simulink subsystem "LaneChangeMetrics"  (R2024b)
settings: Solver=VariableStepAuto  StartTime=0.0  StopTime=10.0  RelTol=1e-3
undefined symbols (not defined in the file): assessment, mapInfo
libraries: simulink x5
settings Model: Creator=The MathWorks, Inc.  LastModifiedBy=The MathWorks, Inc.
settings SolverCC: MaxZcPerStep=1
settings DebuggingCC: UnconnectedInputMsg=warning  UnconnectedOutputMsg=warning  UnconnectedLineMsg=warning  SubsystemReferenceDiagnosticForUnitTest=warning
settings ModelReferenceCC: EnableRefExpFcnMdlSchedulingChecks=on
settings RTWCC: GPUComputeCapability=3.5  DLArmComputeVersion=19.05

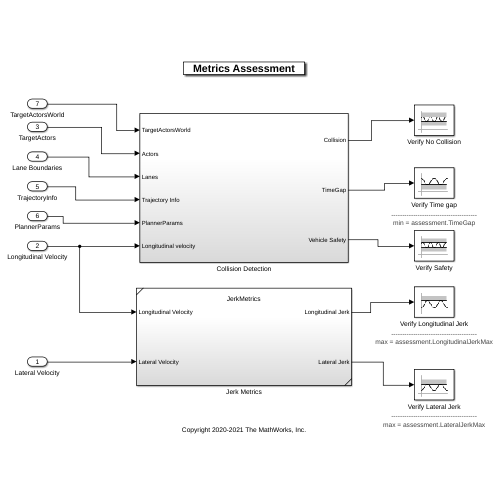
[thumbnail: Simulink's stored preview of the top-level diagram]
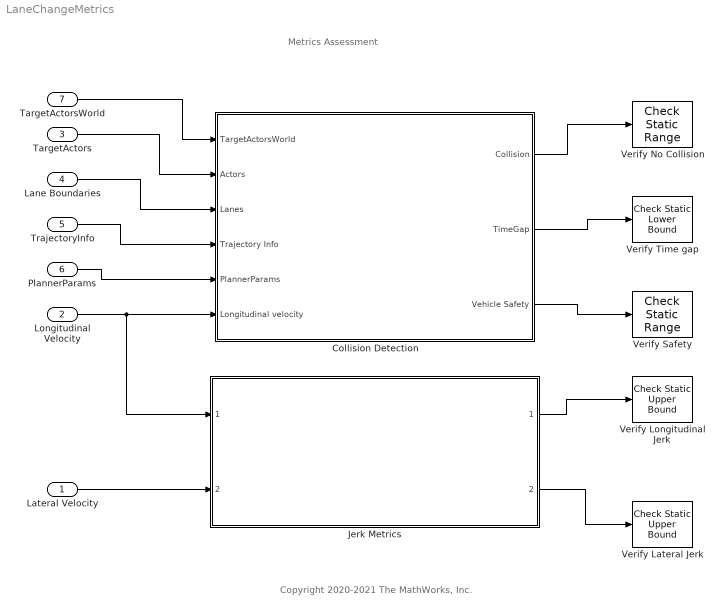
== system LaneChangeMetrics ==
  note: Metrics Assessment
  note: Copyright 2020-2021 The MathWorks, Inc.
  Lateral Velocity : Inport
  Longitudinal Velocity : Inport  Port=2
  TargetActors : Inport  Port=3
  Lane Boundaries : Inport  Port=4
  TrajectoryInfo : Inport  Port=5
  PlannerParams : Inport  Port=6
  TargetActorsWorld : Inport  Port=7
  Collision Detection : Subsystem
  Jerk Metrics : Subsystem  ReferencedSubsystem=JerkMetrics
  Verify Lateral Jerk : simulink/Model Verification/Check Static  Upper Bound  Description=u <= assessment.LateralJerkMax  max=assessment.LateralJerkMax  max_included=on  enabled=on  stopWhenAssertionFail=off  export=off  icon=graphic
      settings: AttributesFormatString=|
      | ---------------------------------------
      | max = %<max>
  Verify Longitudinal Jerk : simulink/Model Verification/Check Static  Upper Bound  Description=u <= assessment.LongitudinalJerkMax  max=assessment.LongitudinalJerkMax  max_included=on  enabled=on  stopWhenAssertionFail=off  export=off  icon=graphic
      settings: AttributesFormatString=|
      | ---------------------------------------
      | max = %<max>
  Verify No Collision : simulink/Model Verification/Check  Static Range  Description=0 <= u <= 0  max=0  max_included=on  min=0  min_included=on  enabled=on  stopWhenAssertionFail=on  export=off  icon=graphic
  Verify Safety : simulink/Model Verification/Check  Static Range  Description=1 <= u <= 1  max=1  max_included=on  min=1  min_included=on  enabled=on  stopWhenAssertionFail=off  export=off  icon=graphic
  Verify Time gap : simulink/Model Verification/Check Static  Lower Bound  Description=assessment.TimeGap <= u  min=assessment.TimeGap  min_included=on  enabled=on  stopWhenAssertionFail=off  export=off  icon=graphic
      settings: AttributesFormatString=|
      | ---------------------------------------
      | min = %<min>
  wires:
  Lateral Velocity/1 -> Jerk Metrics/2
  Jerk Metrics/1 -> Verify Longitudinal Jerk/1
  Jerk Metrics/2 -> Verify Lateral Jerk/1
  TargetActors/1 -> Collision Detection/2(Actors)
  Lane Boundaries/1 -> Collision Detection/3(Lanes)
  Collision Detection/3(Vehicle Safety) -> Verify Safety/1
  Collision Detection/2(TimeGap) -> Verify Time gap/1
  TrajectoryInfo/1 -> Collision Detection/4(Trajectory Info)
  Collision Detection/1(Collision) -> Verify No Collision/1
  PlannerParams/1 -> Collision Detection/5(PlannerParams)
  Longitudinal Velocity/1 -> Collision Detection/6(Longitudinal velocity), Jerk Metrics/1
  TargetActorsWorld/1 -> Collision Detection/1(TargetActorsWorld)

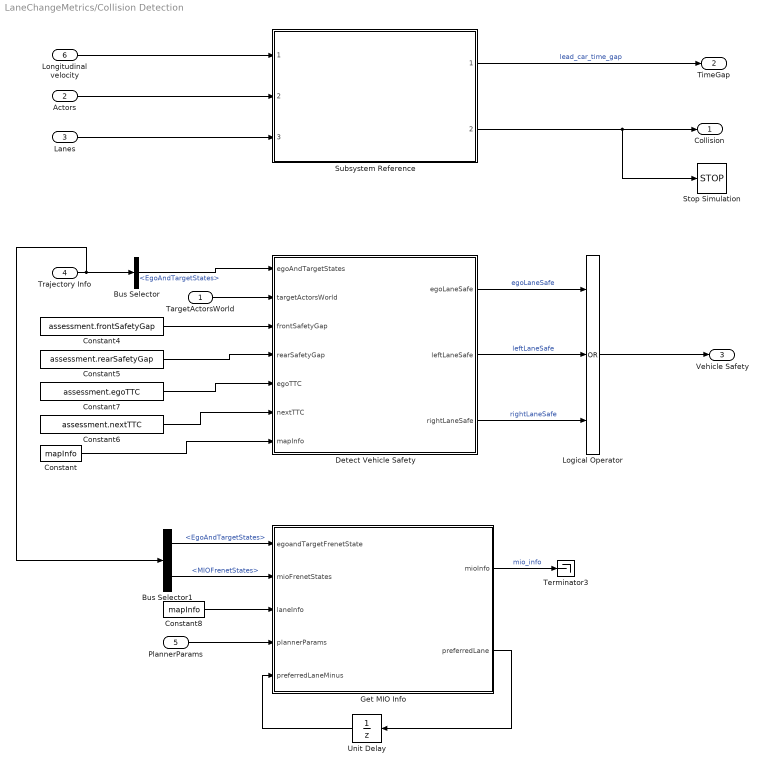
== system LaneChangeMetrics/Collision Detection ==
  TargetActorsWorld : Inport
  Actors : Inport  Port=2
  Lanes : Inport  Port=3
  Trajectory Info : Inport  Port=4
  PlannerParams : Inport  Port=5
  Longitudinal velocity : Inport  Port=6
  Bus Selector : BusSelector  OutputSignals=EgoAndTargetStates
  Bus Selector1 : BusSelector  OutputSignals=EgoAndTargetStates,MIOFrenetStates
  Constant : Constant  Value=mapInfo  OutDataTypeStr=Bus: BusMapInfo
  Constant4 : Constant  Value=assessment.frontSafetyGap
  Constant5 : Constant  Value=assessment.rearSafetyGap
  Constant6 : Constant  Value=assessment.nextTTC
  Constant7 : Constant  Value=assessment.egoTTC
  Constant8 : Constant  Value=mapInfo  OutDataTypeStr=Bus: BusMapInfo
  Detect Vehicle Safety : MATLAB Function  TreatAsAtomicUnit=on
  Get MIO Info : MATLAB Function  TreatAsAtomicUnit=on  mask{outputStructObj=Simulink.Bus.createMATLABStruct('BusMIOInfo')}
      mask prompts: outputStructObj "Output Structure"
  Logical Operator : Logic  Operator=OR  Inputs=3  AllPortsSameDT=off  OutDataTypeStr=boolean
  Stop Simulation : Stop
  Subsystem Reference : Subsystem  ReferencedSubsystem=CollisionDetection
  Terminator3 : Terminator
  Unit Delay : UnitDelay  SampleTime=-1  HasFrameUpgradeWarning=on
  Collision : Outport
  TimeGap : Outport  Port=2
  Vehicle Safety : Outport  Port=3
  wires:
  TargetActorsWorld/1 -> Detect Vehicle Safety/2(targetActorsWorld)
  Constant8/1 -> Get MIO Info/3(laneInfo)
  Bus Selector1/2 -> Get MIO Info/2(mioFrenetStates)  "<MIOFrenetStates>"
  Trajectory Info/1 -> Bus Selector/1, Bus Selector1/1
  Bus Selector1/1 -> Get MIO Info/1(egoandTargetFrenetState)  "<EgoAndTargetStates>"
  Unit Delay/1 -> Get MIO Info/5(preferredLaneMinus)
  Get MIO Info/1(mioInfo) -> Terminator3/1  "mio_info"
  PlannerParams/1 -> Get MIO Info/4(plannerParams)
  Get MIO Info/2(preferredLane) -> Unit Delay/1
  Detect Vehicle Safety/2(leftLaneSafe) -> Logical Operator/2  "leftLaneSafe"
  Detect Vehicle Safety/1(egoLaneSafe) -> Logical Operator/1  "egoLaneSafe"
  Constant4/1 -> Detect Vehicle Safety/3(frontSafetyGap)
  Detect Vehicle Safety/3(rightLaneSafe) -> Logical Operator/3  "rightLaneSafe"
  Constant7/1 -> Detect Vehicle Safety/5(egoTTC)
  Constant/1 -> Detect Vehicle Safety/7(mapInfo)
  Logical Operator/1 -> Vehicle Safety/1
  Constant5/1 -> Detect Vehicle Safety/4(rearSafetyGap)
  Bus Selector/1 -> Detect Vehicle Safety/1(egoAndTargetStates)  "<EgoAndTargetStates>"
  Constant6/1 -> Detect Vehicle Safety/6(nextTTC)
  Subsystem Reference/1 -> TimeGap/1  "lead_car_time_gap"
  Subsystem Reference/2 -> Stop Simulation/1, Collision/1
  Longitudinal velocity/1 -> Subsystem Reference/1
  Actors/1 -> Subsystem Reference/2
  Lanes/1 -> Subsystem Reference/3

== matlab function LaneChangeMetrics/Collision Detection/Detect Vehicle Safety ==
  data: egoAndTargetStates input; targetActorsWorld input; egoLaneSafe output; frontSafetyGap input; rearSafetyGap input; egoTTC input; nextTTC input; mapInfo input; leftLaneSafe output; rightLaneSafe output
function [egoLaneSafe, leftLaneSafe, rightLaneSafe]  = vehicleSafetyDetection(egoAndTargetStates, targetActorsWorld, frontSafetyGap, rearSafetyGap, egoTTC, nextTTC, mapInfo)

egoFrenetState = egoAndTargetStates.EgoFrenetState;

curEgoLane = helperDetectLaneNumber(mapInfo,egoFrenetState(4));
numTargets = targetActorsWorld.NumActors;
targetLanes = zeros(numTargets,1);
targetTTCs = zeros(numTargets,1);
targetRanges = zeros(numTargets,1);
targetVels = zeros(numTargets,1);
targetFront = zeros(numTargets,1);
mioSafe = zeros(numTargets,1);
% egoLaneSafe = 0;
leftLaneSafe = false;
rightLaneSafe = false;


persistent RefPathFrenet 
refPath = mapInfo.GlobalPlanPoints(1:mapInfo.NumGlobalPlanPoints,:);
if isempty(RefPathFrenet)    
    RefPathFrenet = referencePathFrenet(refPath);   
else
    %Check for a change in the reference path
    if ~isequal(RefPathFrenet.Waypoints, refPath) 
        refPathNew = referencePathFrenet(refPath);
        RefPathFrenet.Waypoints = refPathNew.Waypoints;
    end
end

targetStates = zeros(targetActorsWorld.NumActors, 6);
for i=1:numTargets
    targetStates(i,:) = [targetActorsWorld.Actors(i).Position(1:2),...
                       deg2rad(targetActorsWorld.Actors(i).Yaw), 0,...
                       norm(targetActorsWorld.Actors(i).Velocity(1:2)), 0];
    
end
targetFrenetStates = zeros(numTargets, 6);
if(numTargets)
    targetFrenetStates = global2frenet(RefPathFrenet, targetStates);
end
for i = 1:numTargets
        % Get MIO lane
        targetLanes(i) = helperDetectLaneNumber(mapInfo, targetFrenetStates(i,4));        
        
        % Calculate TTC and other attributes of MIOs with ego vehicle
        [targetRanges(i),~,targetVels(i),targetTTCs(i),targetFront(i)] = helperCalculateTTC(egoFrenetState,targetFrenetStates(i,:));
        mioSafe(i) = checkSafety(targetLanes(i),targetRanges(i),targetTTCs(i),targetFront(i),curEgoLane,frontSafetyGap, rearSafetyGap, egoTTC,nextTTC);        
end

% check ego lane
egoLane = targetLanes==curEgoLane;
% disp(mioSafe(egoLane));
egoLaneSafe = isempty(mioSafe(egoLane)) || all(mioSafe(egoLane));


% check left lane
leftLane = targetLanes==(curEgoLane-1);
if curEgoLane>1
    leftLaneSafe = (isempty(mioSafe(leftLane)) || all(mioSafe(leftLane))) ;
end

% check right lane
rightLane = targetLanes==(curEgoLane+1);
if curEgoLane<mapInfo.NumLanes 
    rightLaneSafe = (isempty(mioSafe(rightLane)) || all(mioSafe(rightLane)));
end
end
function isSafe = checkSafety(Lane,Range,TTC,Front,EgoLane,frontSafetyGap,rearSafetyGap,egoTTC,nextTTC)
%checkSafety function checks for safety of current ego lane, and it's
%adjacent lanes.

% default: current lane is unsafe
isSafe = true;

if Front
    SafetyGap = frontSafetyGap;
else
    SafetyGap = rearSafetyGap;
end

if Lane==EgoLane % ego lane
    if Range < SafetyGap || ... % mio is too close?
            (TTC < 0 && ... % mio is approaching
            abs(TTC) < egoTTC) % TTC is too small?
        isSafe = false; % current lane is unsafe
    end
else % left or right lane
    if Range < SafetyGap || ... % mio is too close?
            (TTC < 0 && ... % mio is approaching
            abs(TTC) < nextTTC) % TTC is too small?
        isSafe = false; % current lane is unsafe
    end   
end

end

== matlab function LaneChangeMetrics/Collision Detection/Get MIO Info ==
  data: mioInfo output Bus: BusMIOInfo; egoandTargetFrenetState input; preferredLane output; mioFrenetStates input; laneInfo input; plannerParams input; preferredLaneMinus input; outputStructObj parameter
function [mioInfo, preferredLane] = getMIOInfo(egoandTargetFrenetState,...
                                               mioFrenetStates, laneInfo,...
                                               plannerParams,...
                                               preferredLaneMinus,...
                                               outputStructObj)


% Get ego actor frenet states from EgoAndTargetStates bus structure
egoFrenetState = egoandTargetFrenetState.EgoFrenetState;

[preferredLane, mioInfo]= helperFindPreferredLane(egoFrenetState,...
                                                  mioFrenetStates,...
                                                  laneInfo,plannerParams,...
                                                  preferredLaneMinus,...
                                                  outputStructObj);

end
